simulink model "vehiclecontroller_org"  (Simulink 10.0)
settings: Solver=ode45  StartTime=0.0  StopTime=10.0  RelTol=1e-3  EnableMultiTasking=on
libraries: driveline x4
settings Model: Creator=Elena  LastModifiedBy=bhisma
settings DataIOCC: LimitDataPoints=on
settings DebuggingCC: UnderspecifiedInitializationDetection=Simplified  MergeDetectMultiDrivingBlocksExec=error
settings GRTTargetCC: GeneratePreprocessorConditionals=Disable all  CombineOutputUpdateFcns=on  GRTInterface=off
settings ConfigComp: CovExternalEMLEnable=off
settings SimscapeCC: SimscapeNormalizeSystem=off

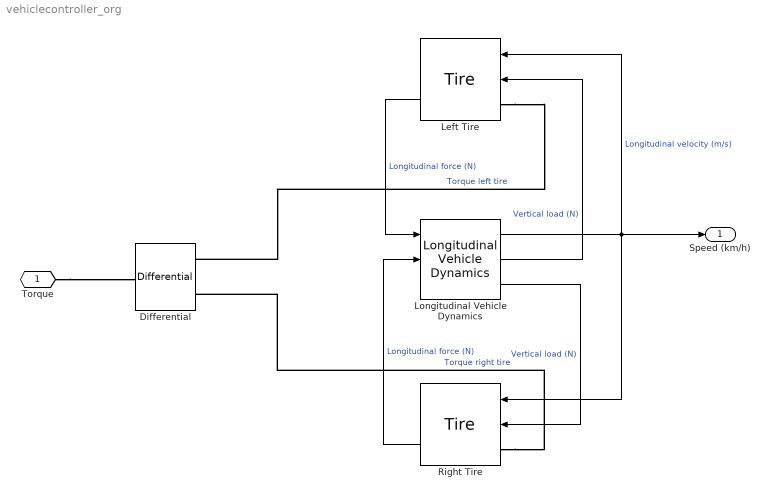
== system vehiclecontroller_org ==
  Differential : driveline/Gears/Differential  R=1  ValidatorFcn=drive_differentialgearblock  SimDrivelineLibraryVersion=1.1
      settings: SourceProductName=Simscape Driveline  SourceProductBaseCode=LD
  Left Tire : driveline/Vehicle Components/Tire  r_e=0.3  F_z=3000  F_x_max=3500  kappa_max=10  sigma_k=0.2
      settings: SourceProductName=Simscape Driveline  SourceProductBaseCode=LD
  Longitudinal Vehicle Dynamics : driveline/Vehicle Components/Longitudinal Vehicle Dynamics  m=1325  a=1.35  b=1.35  h=0.5  FA=2.57  C_d=0.26  v0=0
      settings: SourceProductName=Simscape Driveline  SourceProductBaseCode=LD
  Right Tire : driveline/Vehicle Components/Tire  r_e=0.3  F_z=3000  F_x_max=3500  kappa_max=10  sigma_k=0.2
      settings: SourceProductName=Simscape Driveline  SourceProductBaseCode=LD
  Torque : PMIOPort  Side=Left
  Speed (km/h) : Outport
  wires:
  Left Tire/2 -> Longitudinal Vehicle Dynamics/1  "Longitudinal force (N)"
  Right Tire/2 -> Longitudinal Vehicle Dynamics/2  "Longitudinal force (N)"
  Longitudinal Vehicle Dynamics/2 -> Left Tire/2  "Vertical load (N)"
  Longitudinal Vehicle Dynamics/3 -> Right Tire/2  "Vertical load (N)"
  Longitudinal Vehicle Dynamics/1 -> Left Tire/1, Speed (km/h)/1, Right Tire/1  "Longitudinal velocity (m/s)"
  connections:
  Torque/RConn1 -- Differential/LConn1
  Left Tire/LConn1 -- Differential/RConn1  "Torque left tire"
  Right Tire/LConn1 -- Differential/RConn2  "Torque right tire"
